simulink model "MSDdiscrete"  (R2018a)
settings: Solver=FixedStepDiscrete  StartTime=0.0  StopTime=Tsim  FixedStep=Ts  RelTol=1e-3
values from neighbouring files (symbols this model uses):
  A = [    0    1 ... (first row only)    [massSpringDamper_LQR.m]    (also in msd_least_squares.m = [0    1; -k/m  -c/m]; symbolic_msd.m = [0 1; (-omega_n^2) (-2*omega_n*zeta)])
  Ak = e_ATs    [msd_least_squares.m]    (also in symbolic_msd.m = e_At)
  B = [ 0 ; 1/m]    [massSpringDamper_LQR.m]    (also in msd_least_squares.m; symbolic_msd.m = [0;1/m])
  Bk = mtimes(aux2,B)    [msd_least_squares.m]    (also in symbolic_msd.m)
  dcgain = dcgain(1)    [msd_least_squares.m]
  Ts = 0.5    [massSpringDamper_LQR.m]    (also in msd_least_squares.m; symbolic_msd.m)
  x0 = [0;0]    [massSpringDamper_LQR.m]    (also in msd_least_squares.m)
undefined symbols (not defined in the file or in its folder): Ad, Bd
settings Model: Creator=srivats  LastModifiedBy=srivats

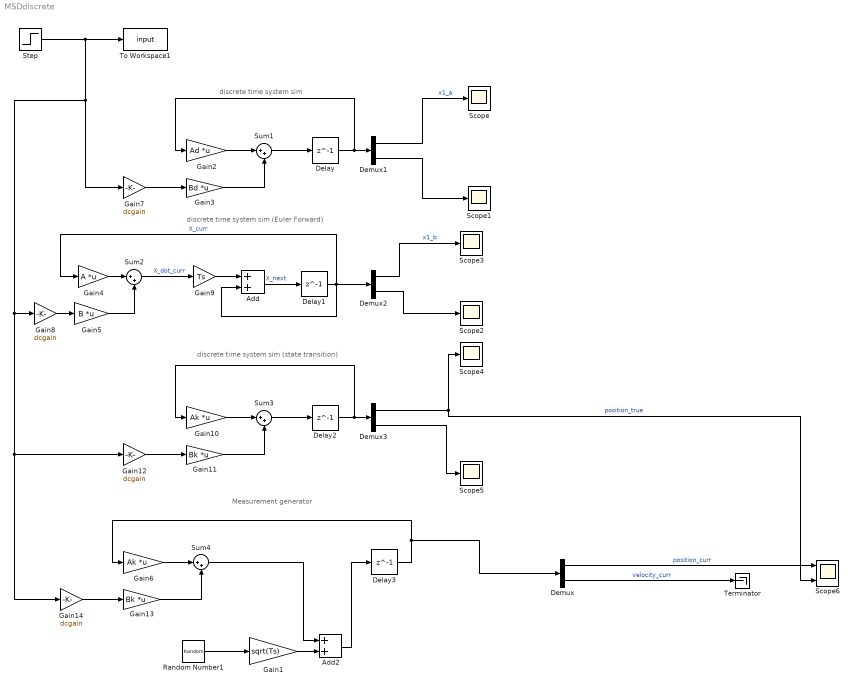
== system MSDdiscrete ==
  note: Measurement generator
  note: discrete time system sim (state transition)
  note: discrete time system sim (Euler Forward)
  note: discrete time system sim
  Add : Sum
  Add2 : Sum
  Delay{,1..3} (4 alike) : Delay  DelayLength=1  InitialCondition=x0  SampleTime=Ts
  Demux{,1..3} (4 alike) : Demux  Outputs=2
  Gain1 : Gain  Gain=sqrt(Ts)
  Gain10 : Gain  Gain=Ak  Multiplication=Matrix(K*u)
  Gain11 : Gain  Gain=Bk  Multiplication=Matrix(K*u)
  Gain{7..8,12,14} (4 alike) : Gain  Gain=dcgain
  Gain13 : Gain  Gain=Bk  Multiplication=Matrix(K*u)
  Gain2 : Gain  Gain=Ad  Multiplication=Matrix(K*u)
  Gain3 : Gain  Gain=Bd  Multiplication=Matrix(K*u)
  Gain4 : Gain  Gain=A  Multiplication=Matrix(K*u)
  Gain5 : Gain  Gain=B  Multiplication=Matrix(K*u)
  Gain6 : Gain  Gain=Ak  Multiplication=Matrix(K*u)
  Gain9 : Gain  Gain=Ts
  Random Number1 : RandomNumber  Variance=0.5  Seed=1  SampleTime=Ts
  Scope{,1..5} (6 alike) : Scope
  Scope6 : Scope  NumInputPorts=3
  Step : Step  SampleTime=Ts
  Sum{1..4} (4 alike) : Sum  Inputs=|++
  Terminator : Terminator
  To Workspace1 : ToWorkspace  VariableName=input  SaveFormat=Timeseries  SampleTime=-1
  wires:
  Gain11/1 -> Sum3/2
  Gain12/1 -> Gain11/1
  Sum3/1 -> Delay2/1
  Sum2/1 -> Gain9/1  "X_dot_curr"
  Gain5/1 -> Sum2/2
  Gain3/1 -> Sum1/2
  Add/1 -> Delay1/1  "X_next"
  Delay1/1 -> Demux2/1, Gain4/1, Add/2  "X_curr"
  Gain7/1 -> Gain3/1
  Gain8/1 -> Gain5/1
  Delay/1 -> Demux1/1, Gain2/1
  Gain2/1 -> Sum1/1
  Demux3/1 -> Scope6/3, Scope4/1  "position_true"
  Gain4/1 -> Sum2/1
  Demux2/1 -> Scope3/1  "x1_b"
  Demux1/1 -> Scope/1  "x1_a"
  Gain9/1 -> Add/1
  Gain10/1 -> Sum3/1
  Sum1/1 -> Delay/1
  Demux3/2 -> Scope5/1
  Demux2/2 -> Scope2/1
  Demux1/2 -> Scope1/1
  Delay2/1 -> Demux3/1, Gain10/1
  Gain6/1 -> Sum4/1
  Gain13/1 -> Sum4/2
  Random Number1/1 -> Gain1/1
  Sum4/1 -> Add2/1
  Delay3/1 -> Gain6/1, Demux/1
  Step/1 -> Gain7/1, Gain14/1, Gain12/1, Gain8/1, To Workspace1/1
  Gain14/1 -> Gain13/1
  Gain1/1 -> Add2/2
  Add2/1 -> Delay3/1
  Demux/1 -> Scope6/1  "position_curr"
  Demux/2 -> Terminator/1  "velocity_curr"
